simulink model "Soal2"  (R2021b)
settings: Solver=VariableStepAuto  StartTime=0.0  StopTime=10.0  RelTol=1e-3
settings Model: Creator=Parsa  LastModifiedBy=Parsa

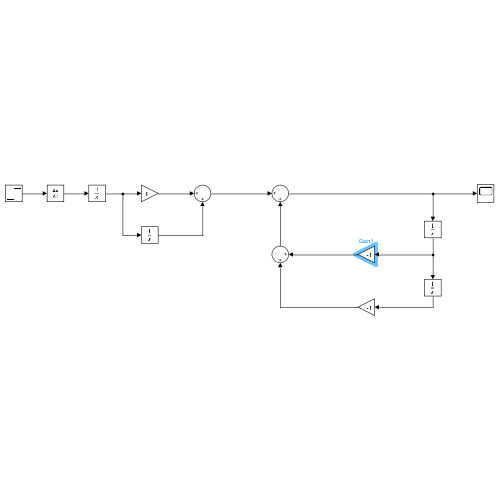
[thumbnail: Simulink's stored preview of the top-level diagram]
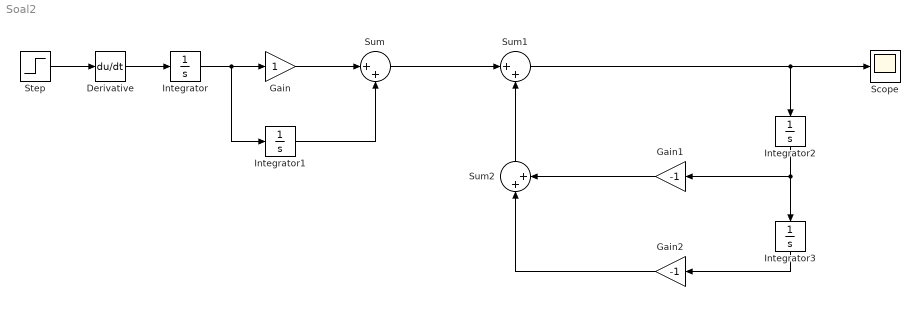
== system Soal2 ==
  Derivative : Derivative
  Gain : Gain
  Gain1 : Gain  Gain=-1
  Gain2 : Gain  Gain=-1
  Integrator{,1..3} (4 alike) : Integrator
  Scope : Scope
  Step : Step  Time=0.001  SampleTime=0
  Sum : Sum  Inputs=|++
  Sum1 : Sum  Inputs=|++
  Sum2 : Sum  Inputs=|++
  wires:
  Integrator/1 -> Integrator1/1, Gain/1
  Gain/1 -> Sum/1
  Integrator1/1 -> Sum/2
  Sum/1 -> Sum1/1
  Integrator2/1 -> Gain1/1, Integrator3/1
  Sum1/1 -> Integrator2/1, Scope/1
  Sum2/1 -> Sum1/2
  Gain1/1 -> Sum2/2
  Integrator3/1 -> Gain2/1
  Gain2/1 -> Sum2/1
  Step/1 -> Derivative/1
  Derivative/1 -> Integrator/1
